simulink model "ipd_controller"  (R2024a)
settings: Solver=VariableStepAuto  StartTime=0.0  StopTime=1  RelTol=1e-3
values from neighbouring files (symbols this model uses):
  a = 8.5879    [cart_ipd_control.m]    (also in ipd_lifted_regulator.m)
  b = 36.081    [cart_ipd_control.m]    (also in ipd_lifted_regulator.m)
  h = 0.02    [cart_ipd_control.m]    (also in ipd_lifted_regulator.m = 0.06)
  kD = (a_2*w-a) / b    (= 2.25637038885)    [cart_ipd_control.m]
  kI = w^3 / b    (= 748.316288351)    [cart_ipd_control.m]
  kP = (a_1*w^2) / b    (= 74.8316288351)    [cart_ipd_control.m]
  t_sim = 0.001    [cart_ipd_control.m]    (also in ipd_lifted_regulator.m)
  x0 = 0.0    (= 0)    [cart_ipd_control.m]    (also in ipd_lifted_regulator.m = [1.5)
  xf = 1.5    [cart_ipd_control.m]
libraries: simulink_extras x2
settings Model: Creator=Fumiya Matsuzaki  LastModifiedBy=Fumiya Matsuzaki

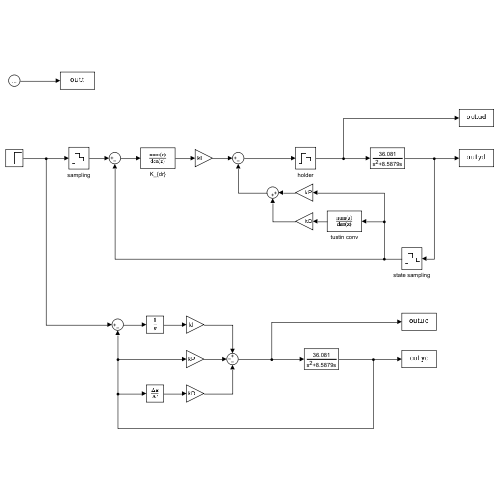
[thumbnail: Simulink's stored preview of the top-level diagram]
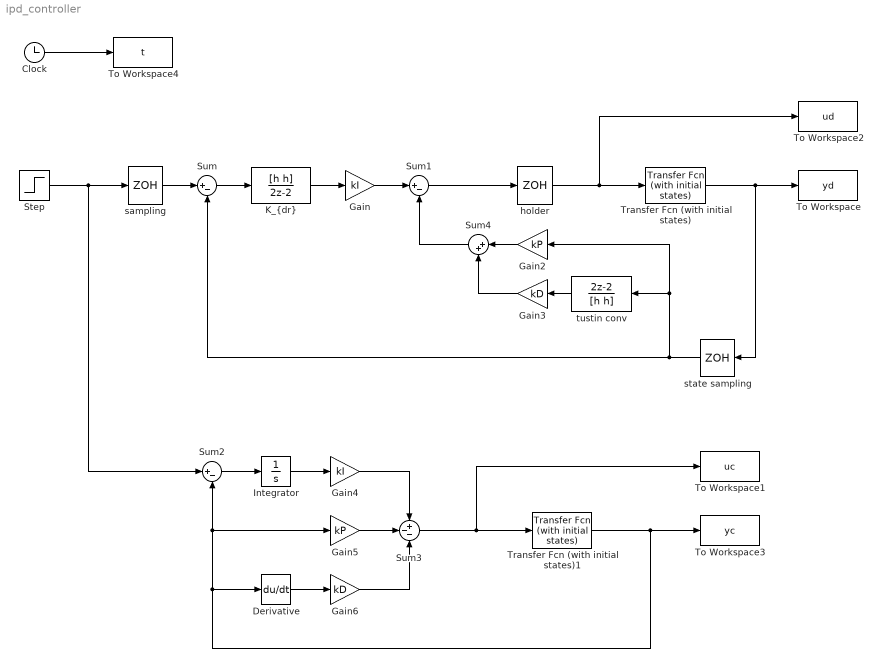
== system ipd_controller ==
  Clock : Clock
  Derivative : Derivative
  Gain : Gain  Gain=kI
  Gain2 : Gain  Gain=kP
  Gain3 : Gain  Gain=kD
  Gain4 : Gain  Gain=kI
  Gain5 : Gain  Gain=kP
  Gain6 : Gain  Gain=kD
  Integrator : Integrator
  "K_{dr}" : DiscreteTransferFcn  Numerator=[h h]  Denominator=[2 -2]  SampleTime=h
  Step : Step  Time=0  After=xf  SampleTime=0
  Sum : Sum  Inputs=|+-
  Sum1 : Sum  Inputs=|+-
  Sum2 : Sum  Inputs=|+-
  Sum3 : Sum  Inputs=+--
  Sum4 : Sum  Inputs=|++
  To Workspace : ToWorkspace  VariableName=yd  SampleTime=t_sim
  To Workspace1 : ToWorkspace  VariableName=uc  SampleTime=t_sim
  To Workspace2 : ToWorkspace  VariableName=ud  SampleTime=t_sim
  To Workspace3 : ToWorkspace  VariableName=yc  SampleTime=t_sim
  To Workspace4 : ToWorkspace  VariableName=t  SampleTime=t_sim
  Transfer Fcn (with initial states) : simulink_extras/Additional Linear/Transfer Fcn (with initial states)  N=[b]  D=[1 a 0]  X0=x0
  Transfer Fcn (with initial states)1 : simulink_extras/Additional Linear/Transfer Fcn (with initial states)  N=[b]  D=[1 a 0]  X0=x0
  holder : ZeroOrderHold  SampleTime=t_sim
  sampling : ZeroOrderHold  SampleTime=h
  state sampling : ZeroOrderHold  SampleTime=h
  tustin conv : DiscreteTransferFcn  Numerator=[2 -2]  Denominator=[h h]  SampleTime=h
  wires:
  Sum3/1 -> Transfer Fcn (with initial states)1/1, To Workspace1/1
  tustin conv/1 -> Gain3/1
  Transfer Fcn (with initial states)1/1 -> To Workspace3/1, Sum2/2, Gain5/1, Derivative/1
  state sampling/1 -> Gain2/1, tustin conv/1, Sum/2
  Gain6/1 -> Sum3/3
  Derivative/1 -> Gain6/1
  Gain4/1 -> Sum3/1
  Gain5/1 -> Sum3/2
  Integrator/1 -> Gain4/1
  Sum/1 -> "K_{dr}"/1
  Sum2/1 -> Integrator/1
  "K_{dr}"/1 -> Gain/1
  Gain/1 -> Sum1/1
  Gain2/1 -> Sum4/1
  Gain3/1 -> Sum4/2
  Sum4/1 -> Sum1/2
  Sum1/1 -> holder/1
  Step/1 -> sampling/1, Sum2/1
  Transfer Fcn (with initial states)/1 -> state sampling/1, To Workspace/1
  holder/1 -> Transfer Fcn (with initial states)/1, To Workspace2/1
  sampling/1 -> Sum/1
  Clock/1 -> To Workspace4/1
